simulink model "lab1schema2rezolvata"  (R2020a)
settings: Solver=VariableStepAuto  StartTime=0.0  StopTime=10.0  RelTol=1e-3
undefined symbols (not defined in the file): sigbuilder_block
settings Model: Creator=Florin Stinga  LastModifiedBy=Alex
settings DataIOCC: ReturnWorkspaceOutputs=off
settings DebuggingCC: ArithmeticOperatorsInVariantConditions=warning
settings SFSimCC: SimUseLocalCustomCode=off  CustomCodeUndefinedFunction=UseInterfaceOnly
settings RTWCC: RTWUseLocalCustomCode=off
settings CodeAppCC: StateflowObjectComments=on

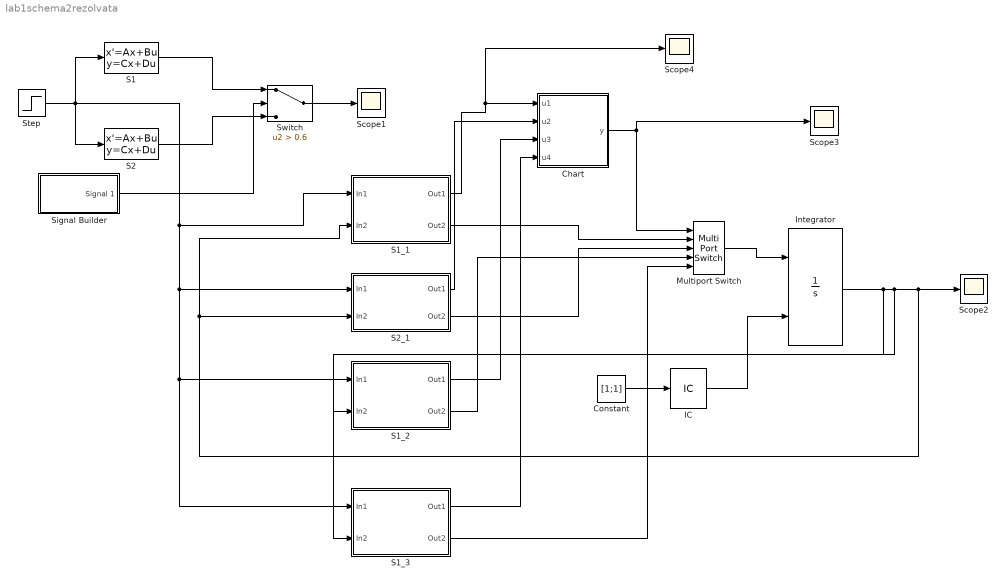
== system lab1schema2rezolvata ==
  Chart : Stateflow chart  TreatAsAtomicUnit=on
  Constant : Constant  Value=[1;1]
  IC : InitialCondition  Value=[1;-1]
  Integrator : Integrator  InitialConditionSource=external
  Multiport Switch : MultiPortSwitch  Inputs=4
  S1 : StateSpace  A=[1 1;-2 -1]  B=[0;1]  C=[2 0]  D=0  InitialCondition=0
  S1_1 : Subsystem
  S1_2 : Subsystem
  S1_3 : Subsystem
  S2 : StateSpace  A=[-1 1;-2 -2]  B=[0;1]  C=[1 1]  D=0  InitialCondition=0
  S2_1 : Subsystem
  Scope{1..4} (4 alike) : Scope
  Signal Builder : Subsystem  Tag=STV Subsys  LoadFcn=sigbuilder_block('load');  StartFcn=sigbuilder_block('start');  StopFcn=sigbuilder_block('stop');  ClipboardFcn=sigbuilder_block('clipboard');  mask(Sigbuilder block){tuvar=[0:10]}
      mask help: Simulink:masks:SigbuilderBlock_MD
      mask init:
      | if ~strcmp(get_param(bdroot(gcbh),'SimulationStatus'),'stopped') tuvar = sigbuilder_block('maskInit'); end
      settings: CopyFcn=sigbuilder_block('copy');  DeleteFcn=sigbuilder_block('delete');  ModelCloseFcn=sigbuilder_block('modelClose');  PreSaveFcn=sigbuilder_block('preSave');  PauseFcn=sigbuilder_block('pause');  ContinueFcn=sigbuilder_block('continue');  NameChangeFcn=sigbuilder_block('namechange');  OpenFcn=sigbuilder_block('open',[71 81.5 550.5 360 ]);  CloseFcn=sigbuilder_block('close');
      mask Display: plot(0, 0, 100, 100,[2, 2, 32, 32, 2], [68, 8, 8, 68, 68],[32, 2], [38, 38], [32, 19, 2],[53, 60, 44], [32, 17, 17, 2],[16, 16, 31, 31]);txt = getActiveGroup(gcbh);text(2, 100, txt,'verticalAlignment', 'top');
  Step : Step  Time=0  SampleTime=0
  Switch : Switch  Criteria=u2 > Threshold  Threshold=0.6
  wires:
  Step/1 -> S1_2/1(In1), S1_3/1(In1), S2_1/1(In1), S1_1/1(In1), S2/1, S1/1
  Switch/1 -> Scope1/1
  S1/1 -> Switch/1
  S2/1 -> Switch/3
  Signal Builder/1(Signal 1) -> Switch/2
  Chart/1(y) -> Multiport Switch/1, Scope3/1
  Multiport Switch/1 -> Integrator/1
  Integrator/1 -> S1_2/2(In2), S1_3/2(In2), S1_1/2(In2), S2_1/2(In2), Scope2/1
  IC/1 -> Integrator/2
  Constant/1 -> IC/1
  S1_1/1(Out1) -> Scope4/1, Chart/1(u1)
  S1_1/2(Out2) -> Multiport Switch/2
  S2_1/1(Out1) -> Chart/2(u2)
  S2_1/2(Out2) -> Multiport Switch/3
  S1_2/1(Out1) -> Chart/3(u3)
  S1_3/1(Out1) -> Chart/4(u4)
  S1_2/2(Out2) -> Multiport Switch/4
  S1_3/2(Out2) -> Multiport Switch/5

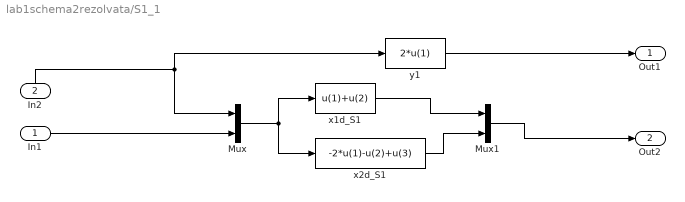
== system lab1schema2rezolvata/S1_1 ==
  In1 : Inport
  In2 : Inport  Port=2
  Mux : Mux  Inputs=2
  Mux1 : Mux  Inputs=2
  x1d_S1 : Fcn  Expr=u(1)+u(2)
  x2d_S1 : Fcn  Expr=-2*u(1)-u(2)+u(3)
  y1 : Fcn  Expr=2*u(1)
  Out1 : Outport
  Out2 : Outport  Port=2
  wires:
  x2d_S1/1 -> Mux1/2
  x1d_S1/1 -> Mux1/1
  Mux1/1 -> Out2/1
  Mux/1 -> x2d_S1/1, x1d_S1/1
  y1/1 -> Out1/1
  In1/1 -> Mux/2
  In2/1 -> Mux/1, y1/1

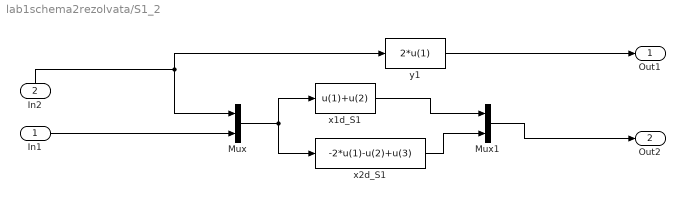
== system lab1schema2rezolvata/S1_2 ==
  In1 : Inport
  In2 : Inport  Port=2
  Mux : Mux  Inputs=2
  Mux1 : Mux  Inputs=2
  x1d_S1 : Fcn  Expr=u(1)+u(2)
  x2d_S1 : Fcn  Expr=-2*u(1)-u(2)+u(3)
  y1 : Fcn  Expr=2*u(1)
  Out1 : Outport
  Out2 : Outport  Port=2
  wires:
  x2d_S1/1 -> Mux1/2
  x1d_S1/1 -> Mux1/1
  Mux1/1 -> Out2/1
  Mux/1 -> x2d_S1/1, x1d_S1/1
  y1/1 -> Out1/1
  In1/1 -> Mux/2
  In2/1 -> Mux/1, y1/1

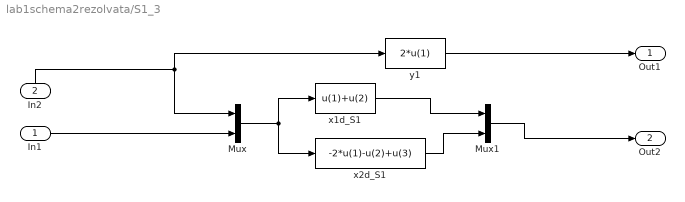
== system lab1schema2rezolvata/S1_3 ==
  In1 : Inport
  In2 : Inport  Port=2
  Mux : Mux  Inputs=2
  Mux1 : Mux  Inputs=2
  x1d_S1 : Fcn  Expr=u(1)+u(2)
  x2d_S1 : Fcn  Expr=-2*u(1)-u(2)+u(3)
  y1 : Fcn  Expr=2*u(1)
  Out1 : Outport
  Out2 : Outport  Port=2
  wires:
  x2d_S1/1 -> Mux1/2
  x1d_S1/1 -> Mux1/1
  Mux1/1 -> Out2/1
  Mux/1 -> x2d_S1/1, x1d_S1/1
  y1/1 -> Out1/1
  In1/1 -> Mux/2
  In2/1 -> Mux/1, y1/1

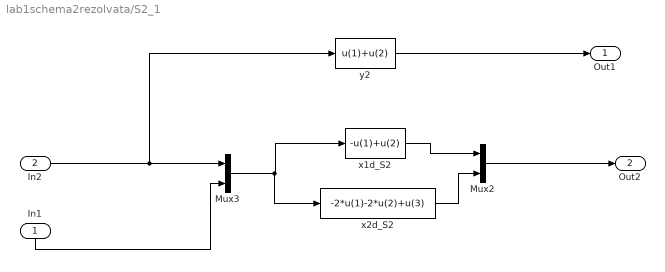
== system lab1schema2rezolvata/S2_1 ==
  In1 : Inport
  In2 : Inport  Port=2
  Mux2 : Mux  Inputs=2
  Mux3 : Mux  Inputs=2
  x1d_S2 : Fcn  Expr=-u(1)+u(2)
  x2d_S2 : Fcn  Expr=-2*u(1)-2*u(2)+u(3)
  y2 : Fcn  Expr=u(1)+u(2)
  Out1 : Outport
  Out2 : Outport  Port=2
  wires:
  In2/1 -> y2/1, Mux3/1
  In1/1 -> Mux3/2
  Mux3/1 -> x2d_S2/1, x1d_S2/1
  x2d_S2/1 -> Mux2/2
  x1d_S2/1 -> Mux2/1
  Mux2/1 -> Out2/1
  y2/1 -> Out1/1

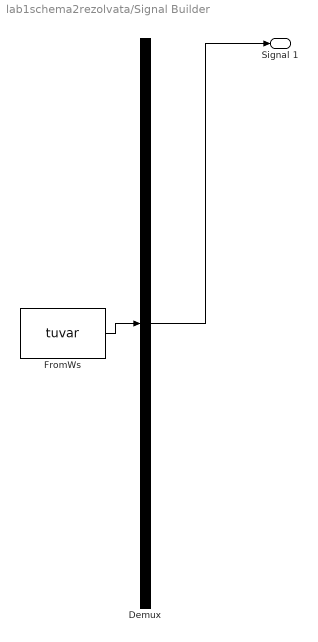
== system lab1schema2rezolvata/Signal Builder ==
  Demux : Demux  Tag=STV Demux  Outputs=1
      settings: DisplayOption=none
  FromWs : FromWorkspace  Tag=STV FromWs  VariableName=tuvar
      SigBuilderData=|
      | common.afterFinalStr = 'Extrapolate'
      | common.sampleTime = 0
      | dataSet.timeRange = [0 10]
      | dataSet.name = 'Group 1'
      | sbobj.Groups.Name = 'Group 1'
      | sbobj.Groups.Signals.Name = 'Signal 1'
      | sbobj.Groups.Signals.XData = [0 1.52 1.52 2.16 2.16 2.86 2.86 4 4 6 6 8.24 8.24 10]
      | sbobj.Groups.Signals.YData = [0.2 0.2 0.69 0.69 0.5 0.5 0.315 0.315 0.67 0.67 0.335 0.335 0.26 0.26]
  Signal 1 : Outport  Tag=STV Outport
  wires:
  Demux/1 -> Signal 1/1
  FromWs/1 -> Demux/1

== stateflow chart lab1schema2rezolvata/Chart ==
  settings: executeAtInitialization=1
  state S1
    en:y=1;c = 0;
    du:c = c + 1;
    exit:
  state S2
    en:y=2; c =0;
    du:c = c + 1;
  state S4
    en:y=1;c = 0;
    du:c = c + 1;
    exit:
  state S3
    en:y=2; c =0;
    du:c = c + 1;
  (default) -> S1
  S1 -> S2 : [u1>=0.3&&c>10]
  S2 -> S1 [order 2] : [u2<1.5&&c>10]
  S2 -> S3 [order 1] : [u3<0.3&&c>10]
  S4 -> S1 : [u1<0.3&&c>10]
  S3 -> S4 : [u4<0.3&&c>10]
  data: y output size=1; u1 input size=1; u2 input size=1; u3 input size=1; c local; u4 input size=1
